simulink model "MPPT_using_Current_fed_Push_pull"  (R2019a)
settings: Solver=FixedStepAuto  StartTime=0.0  StopTime=2.4  FixedStep=Tss  RelTol=1e-3
undefined symbols (not defined in the file): Cin, Tpwm, Tss
libraries: powerlib x29, eePwmGenerator x2, re_lib x1, simulink x1
settings Model: Creator=asus  LastModifiedBy=asus

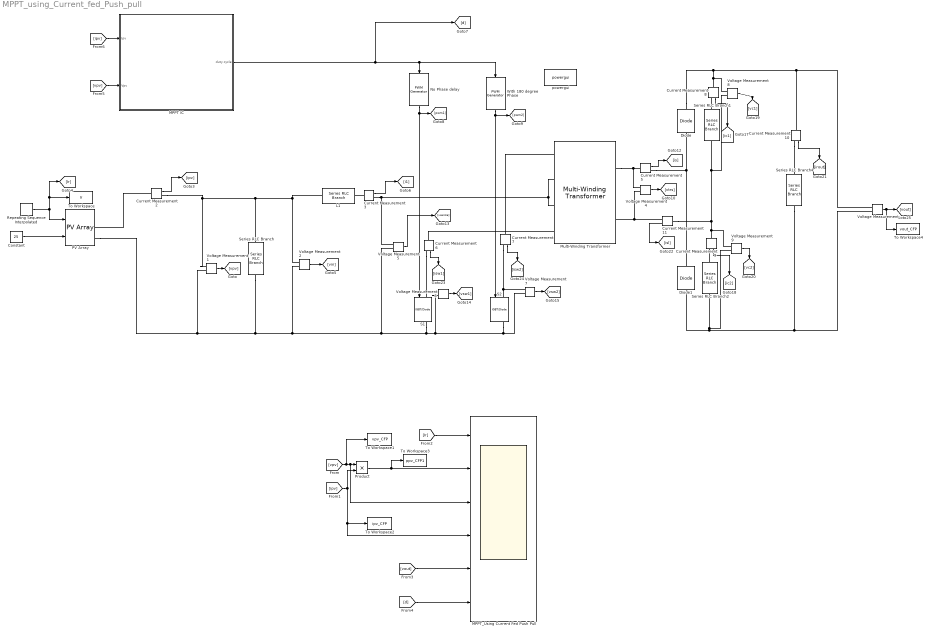
== system MPPT_using_Current_fed_Push_pull ==
  Constant : Constant  Value=25
  Current Measurement{2..3,5..11} (9 alike) : powerlib/Measurements/Current Measurement  PhasorSimulation=off  OutputType=Complex  PSBequivalent=0
      settings: SourceProductName=Simscape Electrical
  Diode : powerlib/Power Electronics/Diode  Ron=1e-6  Lon=1e-9  Vf=0  IC=0  UseSnubber=0  Rs=500  Cs=250e-9  Measurements=off
      settings: SourceProductName=Simscape Electrical
  Diode1 : powerlib/Power Electronics/Diode  Ron=1e-6  Lon=1e-9  Vf=0  IC=0  UseSnubber=0  Rs=500  Cs=250e-9  Measurements=off
      settings: SourceProductName=Simscape Electrical
  L1 : powerlib/Elements/Series RLC Branch  LConnTagsString=__new0  RConnTagsString=__new0  BranchType=L  Resistance=1  Inductance=400e-6  SetiL0=off  InitialCurrent=0  Capacitance=Cin  Setx0=off  InitialVoltage=0  Measurements=None
      settings: SourceProductName=Simscape Electrical
  MPPT IC : Subsystem
  MPPT_Using Current Fed Push Pull : Scope  NumInputPorts=6
  Multi-Winding Transformer : powerlib/Elements/Multi-Winding Transformer  LeftWindings=2  RightWindings=1  TappedWindings=no taps  NumberOfTaps=2  SetSaturation=off  Hysteresis=off  DataFile='hysteresis.mat'  Measurements=None  UNITS=SI  NominalPower=[250 1/Tpwm]  NominalVoltages=[ 100 100 400]  WindingResistances=[0 0 0]  WindingInductances=[0 0 0]  Rm=5.5296e+06  Lm=0.046688  Saturation=[0 0;0.062501 0.029181;26.042 0.036962]  BreakLoop=off  DiscreteSolver=Trapezoidal iterative  DataType=on  InitialFlux=0  TransfoNumber=1
      settings: SourceProductName=Simscape Electrical  SourceProductBaseCode=PS
  No Phase delay : eePwmGenerator/PWM Generator  CarrCount=Up  Tper=Tpwm  Ts=Tss
      settings: SourceProductName=Simscape Electrical
  PV Array : re_lib/Solar/PV Array  Npar=1  Nser=1  PlotType=array @ 25 deg.C & specified irradiances  S_vec="[ 1000 800 500  300 100 ]"  Temp_C_vec="[ 45 25  ]"  ModuleName=1Soltech 1STH-215-P  PlotWhenSelected=off  Pm=213.15  Ncell=60  Voc=36.3  Isc=7.84  Vm=29  Im=7.35  beta_Voc_pc=-0.36099  alpha_Isc_pc=0.102  beta_Voc=-0.13104  alpha_Isc=0.007997  IL=7.8649  I0=2.9259e-10  nI=0.98117  Rsh=313.3991  Rs=0.39383  BAL=on  Tc=1e-6  Tfilter=5e-5
      settings: SourceProductName=Simscape Electrical
  Product : Product
  Repeating Sequence Interpolated : simulink/Sources/Repeating Sequence Interpolated  OutValues=[800 800 1000 1000 500 500].'  TimeValues=[0 .8 .80001 1.6 1.60001 2.4].'  LookUpMeth=Interpolation-Use End Values  tsamp=0.01  OutMin=[]  OutMax=[]  OutDataTypeStr=double  OutputDataTypeScalingMode=double  OutDataType=fixdt(0,8)  OutScaling=2^-10
  S1 : powerlib/Power Electronics/IGBT//Diode  Ron=1e-3  Rs=1e5  Cs=inf  Measurements=on
      settings: SourceProductName=Simscape Electrical
  S2 : powerlib/Power Electronics/IGBT//Diode  Ron=1e-3  Rs=1e5  Cs=inf  Measurements=on
      settings: SourceProductName=Simscape Electrical
  Series RLC Branch : powerlib/Elements/Series RLC Branch  LConnTagsString=__new0  RConnTagsString=__new0  BranchType=RC  Resistance=1e-3  Inductance=1e-3  SetiL0=off  InitialCurrent=0  Capacitance=100e-6  Setx0=off  InitialVoltage=0  Measurements=None
      settings: SourceProductName=Simscape Electrical
  Series RLC Branch1 : powerlib/Elements/Series RLC Branch  LConnTagsString=__new0  RConnTagsString=__new0  BranchType=C  Resistance=1  Inductance=1e-3  SetiL0=off  InitialCurrent=0  Capacitance=20e-6  Setx0=off  InitialVoltage=0  Measurements=Branch voltage
      settings: SourceProductName=Simscape Electrical
  Series RLC Branch2 : powerlib/Elements/Series RLC Branch  LConnTagsString=__new0  RConnTagsString=__new0  BranchType=C  Resistance=1  Inductance=1e-3  SetiL0=off  InitialCurrent=0  Capacitance=20e-6  Setx0=off  InitialVoltage=0  Measurements=Branch voltage
      settings: SourceProductName=Simscape Electrical
  Series RLC Branch4 : powerlib/Elements/Series RLC Branch  LConnTagsString=__new0  RConnTagsString=__new0  BranchType=R  Resistance=1000  Inductance=1e-3  SetiL0=off  InitialCurrent=0  Capacitance=470e-6  Setx0=off  InitialVoltage=0  Measurements=None
      settings: SourceProductName=Simscape Electrical
  To Workspace : ToWorkspace  VariableName=Ir  SaveFormat=Timeseries  SampleTime=Tss
  To Workspace1 : ToWorkspace  VariableName=vpv_CFP  SaveFormat=Timeseries  SampleTime=Tss
  To Workspace2 : ToWorkspace  VariableName=ipv_CFP  SaveFormat=Timeseries  SampleTime=Tss
  To Workspace3 : ToWorkspace  VariableName=ppv_CFP1  SaveFormat=Timeseries  SampleTime=Tss
  To Workspace4 : ToWorkspace  VariableName=vout_CFP  SaveFormat=Timeseries  SampleTime=Tss
  Voltage Measurement{,1..2,4..9} (9 alike) : powerlib/Measurements/Voltage Measurement  PhasorSimulation=off  OutputType=Complex  PSBequivalent=0
      settings: SourceProductName=Simscape Electrical
  With 180 degree Phase : eePwmGenerator/PWM Generator  CarrCount=Up  Tper=Tpwm  Ts=Tss
      link override Carrier counter: Tdelay=Tper*0.5
      settings: SourceProductName=Simscape Electrical
  powergui : powerlib/powergui  Priority=1  SimulationMode=Discrete  SampleTime=Tss  frequency=60  Iterations=50  frequencyindice=0  Pbase=100e6  ErrMax=1e-4  UnitsV=kV  UnitsW=MW  buscounter=0  FunctionMessages=off  echomessages=off  EnableUseOfTLC=off  CurrentSourceSwitches=off  DisableSnubberDevices=off  DisableRonSwitches=off  DisableVfSwitches=off  DisplayEquations=off  AutomaticDiscreteSolvers=off  SolverType=Tustin/Backward Euler (TBE)  Interpol=off  ExternalGateDelay=off  methode=off  Ts=100  x0status=blocks  SPID=on  SwTol=0  HookPort=off  NonlinearTolerance=0  nMaxIteration=15  ContinueOnMaxIteration=off  RestoreLinks=warning  ResistiveCurrentMeasurement=off  Frange=[0:2:500]  Ylog=off  Xlog=on  ShowGrid=off  save=off  variable=ZData  structure=0  ZoomFFT=off  StartTime=0.0  cycles=1  DisplayStyle=1  fundamental=60  FreqAxis=off  MaxFrequency=1000  frequencyindicesteady=1  RmsSteady=1  display=off
      settings: SourceProductName=Simscape Electrical
  wires:
  Repeating Sequence Interpolated/1 -> To Workspace/1, [Ir], PV Array/1
  Constant/1 -> PV Array/2
  [vpv] -> MPPT IC/2(Vpv)
  With 180 degree Phase/1 -> [pwm2], S2/1
  [ipv] -> MPPT IC/1(Ipv)
  Current Measurement2/1 -> [ipv]
  MPPT IC/1(duty cycle) -> [d], No Phase delay/1, With 180 degree Phase/1
  Voltage Measurement1/1 -> [vpv]
  Voltage Measurement5/1 -> [vcentre]
  Current Measurement8/1 -> [ic1]
  Current Measurement7/1 -> [isw2]
  Current Measurement10/1 -> [irout]
  Voltage Measurement9/1 -> [vc2]
  Voltage Measurement2/1 -> [vin]
  Current Measurement9/1 -> [ic2]
  Current Measurement3/1 -> [i1]
  Current Measurement6/1 -> [isw1]
  Voltage Measurement/1 -> To Workspace4/1, [vout]
  Voltage Measurement4/1 -> [vtrs]
  Voltage Measurement6/1 -> [vsw1]
  Voltage Measurement7/1 -> [vsw2]
  Voltage Measurement8/1 -> [vc1]
  Current Measurement11/1 -> [isl]
  Current Measurement5/1 -> [is]
  No Phase delay/1 -> [pwm1], S1/1
  [Ir] -> MPPT_Using Current Fed Push Pull/1
  [vpv] -> To Workspace1/1, MPPT_Using Current Fed Push Pull/3, Product/1
  [ipv] -> Product/2, To Workspace2/1, MPPT_Using Current Fed Push Pull/4
  Product/1 -> To Workspace3/1, MPPT_Using Current Fed Push Pull/2
  [vout] -> MPPT_Using Current Fed Push Pull/5
  [d] -> MPPT_Using Current Fed Push Pull/6
  connections:
  Voltage Measurement2/LConn1 -- L1/LConn1 -- Voltage Measurement1/LConn1 -- Current Measurement2/RConn1 -- Series RLC Branch/LConn1
  Current Measurement2/LConn1 -- PV Array/RConn1
  Multi-Winding Transformer/LConn3 -- Multi-Winding Transformer/LConn2 -- Voltage Measurement5/LConn1 -- Current Measurement3/RConn1
  Voltage Measurement9/LConn2 -- Voltage Measurement/LConn2 -- Series RLC Branch4/RConn1 -- Diode1/LConn1 -- Series RLC Branch2/RConn1
  Multi-Winding Transformer/RConn2 -- Voltage Measurement4/LConn2 -- Current Measurement11/RConn1
  Series RLC Branch1/RConn1 -- Voltage Measurement8/LConn2 -- Current Measurement11/LConn1 -- Current Measurement9/LConn1 -- Voltage Measurement9/LConn1
  Voltage Measurement1/LConn2 -- Series RLC Branch/RConn1 -- Voltage Measurement2/LConn2 -- S1/RConn1 -- S2/RConn1 -- Voltage Measurement7/LConn2 -- Voltage Measurement6/LConn2 -- Voltage Measurement5/LConn2 -- PV Array/RConn2
  Multi-Winding Transformer/RConn1 -- Current Measurement5/LConn1 -- Voltage Measurement4/LConn1
  Diode/RConn1 -- Current Measurement8/LConn1 -- Voltage Measurement8/LConn1 -- Current Measurement10/LConn1 -- Voltage Measurement/LConn1
  Voltage Measurement7/LConn1 -- S2/LConn1 -- Current Measurement7/RConn1
  Diode1/RConn1 -- Current Measurement5/RConn1 -- Diode/LConn1
  Current Measurement6/RConn1 -- S1/LConn1 -- Voltage Measurement6/LConn1
  Current Measurement7/LConn1 -- Multi-Winding Transformer/LConn1
  Current Measurement10/RConn1 -- Series RLC Branch4/LConn1
  Current Measurement3/LConn1 -- L1/RConn1
  Current Measurement6/LConn1 -- Multi-Winding Transformer/LConn4
  Series RLC Branch1/LConn1 -- Current Measurement8/RConn1
  Series RLC Branch2/LConn1 -- Current Measurement9/RConn1

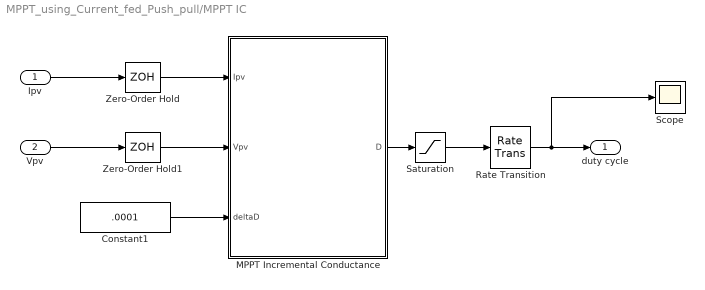
== system MPPT_using_Current_fed_Push_pull/MPPT IC ==
  Ipv : Inport
  Vpv : Inport  Port=2
  Constant1 : Constant  Value=.0001
  MPPT Incremental Conductance : Stateflow chart  BlockKeywords=__PRM__SERIALIZED__DATA__:Stateflow Chart,Stateflow Diagram  TreatAsAtomicUnit=on
  Rate Transition : RateTransition
  Saturation : Saturate  UpperLimit=0.95  LowerLimit=.55
  Scope : Scope
  Zero-Order Hold : ZeroOrderHold  SampleTime=4*Tpwm
  Zero-Order Hold1 : ZeroOrderHold  SampleTime=4*Tpwm
  duty cycle : Outport
  wires:
  Constant1/1 -> MPPT Incremental Conductance/3(deltaD)
  Saturation/1 -> Rate Transition/1
  Rate Transition/1 -> Scope/1, duty cycle/1
  MPPT Incremental Conductance/1(D) -> Saturation/1
  Zero-Order Hold1/1 -> MPPT Incremental Conductance/2(Vpv)
  Zero-Order Hold/1 -> MPPT Incremental Conductance/1(Ipv)
  Ipv/1 -> Zero-Order Hold/1
  Vpv/1 -> Zero-Order Hold1/1

== stateflow chart MPPT_using_Current_fed_Push_pull/MPPT IC/MPPT Incremental Conductance ==
  state SampleAndCalculate
    entry:
    dV=Vpv-Vpre;
    dI=Ipv-Ipre;
  state Init
    entry:
    Vpre=0;
    Ipre=0;
    D=0.9;
  state Decrease_Voltage
    entry:
    D=D+deltaD
  state Increase_Voltage
    entry:
    D=D-deltaD;
  state Increase_Voltage1
    entry:
    D=D-deltaD;
  state Decrease_Voltage1
    entry:
    D=D+deltaD;
  state RETURN
    entry:
    Vpre=Vpv;
    Ipre=Ipv;
  (junction 33) -> SampleAndCalculate
  (default) -> Init
  Init -> SampleAndCalculate
  SampleAndCalculate -> (junction 3) [order 1] : [dV~=0]
  SampleAndCalculate -> (junction 4) [order 2]
  (junction 3) -> (junction 24) [order 3]
  (junction 4) -> (junction 49) [order 3]
  (junction 4) -> Increase_Voltage1 [order 1] : [dI>0]
  (junction 3) -> Increase_Voltage [order 1] : [(Vpv*(dI/dV)+Ipv)>0]
  (junction 3) -> Decrease_Voltage [order 2] : [(Vpv*(dI/dV)+Ipv)<0]
  (junction 4) -> Decrease_Voltage1 [order 2] : [dI<0]
  RETURN -> (junction 33)
  (junction 49) -> RETURN
  (junction 24) -> RETURN
  Increase_Voltage -> RETURN
  Increase_Voltage1 -> RETURN
  Decrease_Voltage1 -> RETURN
  Decrease_Voltage -> RETURN
  data: Ipv input; Vpv input; deltaD input; Ipre local; dV local; dI local; Vpre local; D output
